simulink model "Task_Simulink"  (R2024a)
settings: Solver=VariableStepAuto  StartTime=0.0  StopTime=10.0  RelTol=1e-3
libraries: cstblocks x10
settings Model: Creator=PMYLS  LastModifiedBy=PMYLS

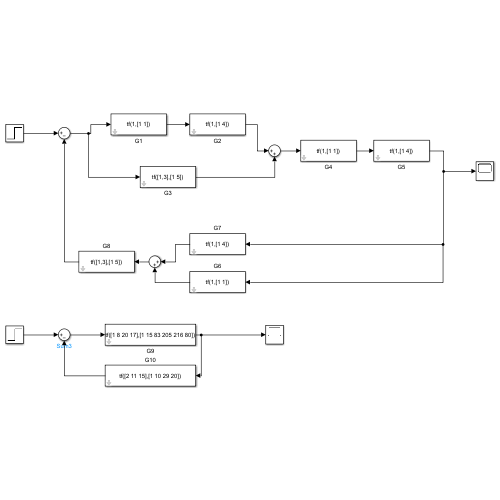
[thumbnail: Simulink's stored preview of the top-level diagram]
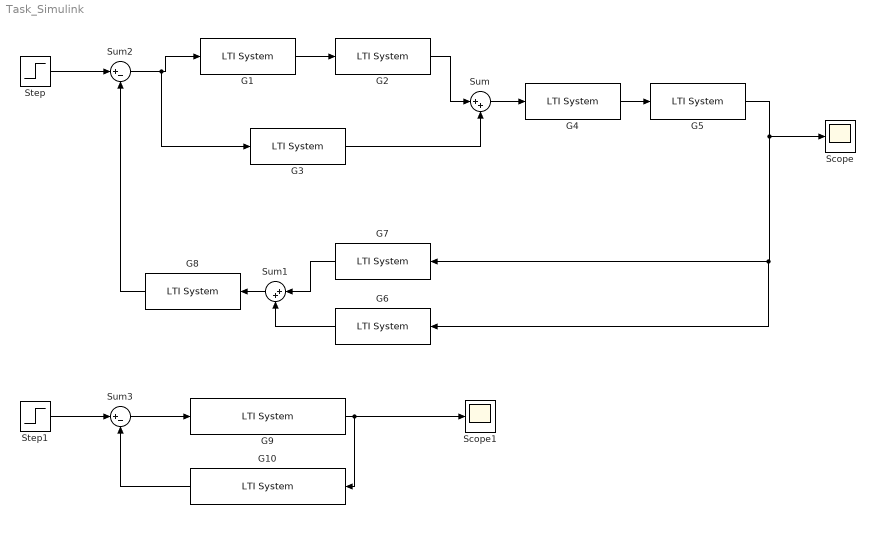
== system Task_Simulink ==
  G1 : cstblocks/LTI System  sys=tf(1,[1 1])  IC=[]  PadeOrder=0
  G10 : cstblocks/LTI System  sys=tf([2 11 15],[1 10 29 20])  IC=[]  PadeOrder=0
  G2 : cstblocks/LTI System  sys=tf(1,[1 4])  IC=[]  PadeOrder=0
  G3 : cstblocks/LTI System  sys=tf([1,3],[1 5])  IC=[]  PadeOrder=0
  G4 : cstblocks/LTI System  sys=tf(1,[1 1])  IC=[]  PadeOrder=0
  G5 : cstblocks/LTI System  sys=tf(1,[1 4])  IC=[]  PadeOrder=0
  G6 : cstblocks/LTI System  sys=tf(1,[1 1])  IC=[]  PadeOrder=0
  G7 : cstblocks/LTI System  sys=tf(1,[1 4])  IC=[]  PadeOrder=0
  G8 : cstblocks/LTI System  sys=tf([1,3],[1 5])  IC=[]  PadeOrder=0
  G9 : cstblocks/LTI System  sys=tf([1 8 20 17],[1 15 83 205 216 80])  IC=[]  PadeOrder=0
  Scope : Scope
  Scope1 : Scope
  Step : Step  SampleTime=0
  Step1 : Step  SampleTime=0
  Sum : Sum  Inputs=|++
  Sum1 : Sum  Inputs=|++
  Sum2 : Sum  Inputs=|+-
  Sum3 : Sum  Inputs=|+-
  wires:
  G1/1 -> G2/1
  G2/1 -> Sum/1
  G3/1 -> Sum/2
  G4/1 -> G5/1
  Sum/1 -> G4/1
  Sum1/1 -> G8/1
  G7/1 -> Sum1/1
  G6/1 -> Sum1/2
  G5/1 -> G6/1, G7/1, Scope/1
  Step/1 -> Sum2/1
  G8/1 -> Sum2/2
  Sum2/1 -> G3/1, G1/1
  Step1/1 -> Sum3/1
  Sum3/1 -> G9/1
  G10/1 -> Sum3/2
  G9/1 -> G10/1, Scope1/1
